simulink model "partB"  (R2018b)
settings: Solver=VariableStepAuto  StartTime=0.0  StopTime=100  RelTol=1e-3
libraries: simulink x2
settings Model: Creator=ms18975  LastModifiedBy=shins

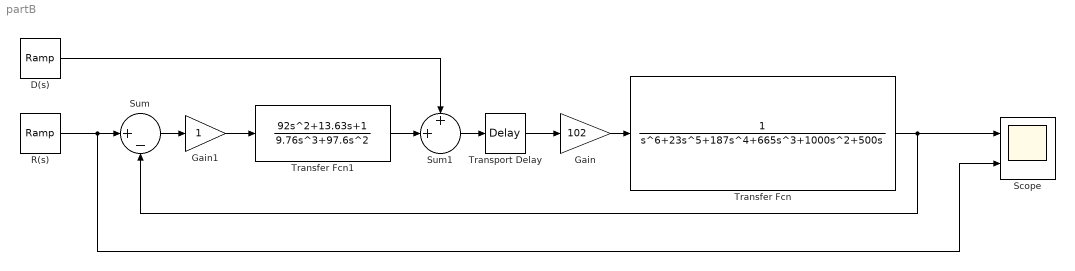
== system partB ==
  D(s) : simulink/Sources/Ramp  slope=0.25  start=50  InitialOutput=0
  Gain : Gain  Gain=102
  Gain1 : Gain
  R(s) : simulink/Sources/Ramp  slope=1  start=0  InitialOutput=0
  Scope : Scope  NumInputPorts=2
  Sum : Sum  Inputs=|+-
  Sum1 : Sum  Inputs=++|
  Transfer Fcn : TransferFcn  Denominator=[1 23 187 665 1000 500 0]
  Transfer Fcn1 : TransferFcn  Numerator=[92 13.63 1]  Denominator=[9.76 97.6 0 0]
  Transport Delay : TransportDelay  DelayTime=0.2
  wires:
  R(s)/1 -> Scope/2, Sum/1
  Transport Delay/1 -> Gain/1
  Sum/1 -> Gain1/1
  Transfer Fcn1/1 -> Sum1/2
  Transfer Fcn/1 -> Scope/1, Sum/2
  Sum1/1 -> Transport Delay/1
  D(s)/1 -> Sum1/1
  Gain/1 -> Transfer Fcn/1
  Gain1/1 -> Transfer Fcn1/1
